simulink model "model1"  (R2020a)
settings: Solver=VariableStepAuto  StartTime=0.0  StopTime=10.0  RelTol=1e-3
settings Model: Creator=hp  LastModifiedBy=hp

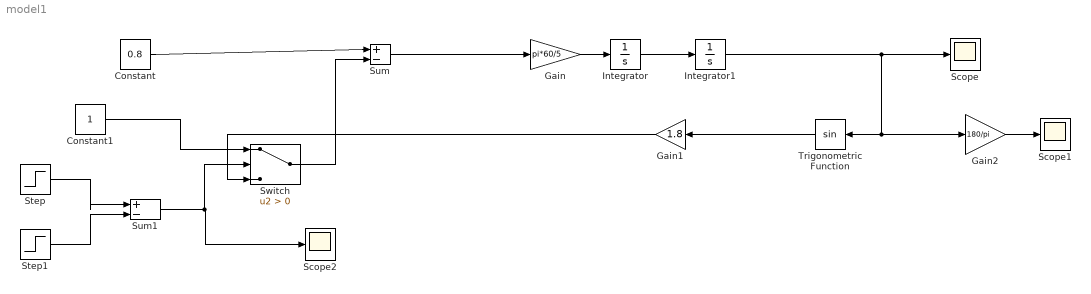
== system model1 ==
  Constant : Constant  Value=0.8
  Constant1 : Constant
  Gain : Gain  Gain=pi*60/5
  Gain1 : Gain  Gain=1.8
  Gain2 : Gain  Gain=180/pi
  Integrator : Integrator
  Integrator1 : Integrator  InitialCondition=26.38*pi/180
  Scope : Scope
  Scope1 : Scope
  Scope2 : Scope
  Step : Step  SampleTime=0
  Step1 : Step  Time=1.26  SampleTime=0
  Sum : Sum  Inputs=|+-
  Sum1 : Sum  Inputs=|+-
  Switch : Switch  Criteria=u2 > Threshold
  Trigonometric Function : Trigonometry
  wires:
  Constant/1 -> Sum/1
  Sum/1 -> Gain/1
  Gain/1 -> Integrator/1
  Integrator/1 -> Integrator1/1
  Integrator1/1 -> Trigonometric Function/1, Gain2/1, Scope/1
  Trigonometric Function/1 -> Gain1/1
  Gain2/1 -> Scope1/1
  Step/1 -> Sum1/1
  Step1/1 -> Sum1/2
  Switch/1 -> Sum/2
  Constant1/1 -> Switch/1
  Sum1/1 -> Switch/2, Scope2/1
  Gain1/1 -> Switch/3
